simulink model "PID_discrete"  (R2019b)
settings: Solver=ode3  StartTime=0.0  StopTime=4  FixedStep=0.001  RelTol=1e-3
undefined symbols (not defined in the file): DiscIntNeverNeededParam
libraries: STLLib x15, discretizing x2
settings Model: Creator=balsi  LastModifiedBy=yuxia
settings DataIOCC: LimitDataPoints=on  SaveFormat=Array  ReturnWorkspaceOutputs=off
settings OptimizationCC: LifeSpan=inf
settings DebuggingCC: SFUnexpectedBacktrackingDiag=warning  SFNoUnconditionalDefaultTransitionDiag=warning  SFExecutionAtInitializationDiag=none  ArithmeticOperatorsInVariantConditions=warning
settings HardwareCC: ProdBitPerPointer=32  ProdBitPerSizeT=32  ProdBitPerPtrDiffT=32  ProdLargestAtomicFloat=None  ProdIntDivRoundTo=Undefined  ProdEndianess=Unspecified  ProdWordSize=32  ProdHWDeviceType=32-bit Generic
settings ModelReferenceCC: PropagateSignalLabelsOutOfModel=off
settings SFSimCC: SimUseLocalCustomCode=off  CustomCodeUndefinedFunction=UseInterfaceOnly
settings RTWCC: RTWUseLocalCustomCode=off
settings CodeAppCC: StateflowObjectComments=on
settings GRTTargetCC: TargetLangStandard=C89/C90 (ANSI)  GeneratePreprocessorConditionals=Disable all
settings ConfigComp: CovMetricSettings=dw  CovHtmlReporting=on  CovSaveCumulativeToWorkspaceVar=on  CovSaveSingleToWorkspaceVar=on  CovExternalEMLEnable=off

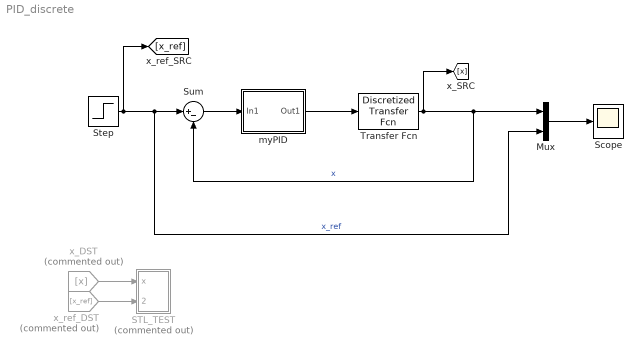
== system PID_discrete ==
  Mux : Mux  Inputs=2
  STL_TEST : Subsystem  Commented=on
  Scope : Scope
  Step : Step  After=10  SampleTime=0.01  mask(DiscretizedSource){}
      mask init:
      | %zoh
  Sum : Sum  Inputs=|+-
  Transfer Fcn : discretizing/Discretized Transfer Fcn  Numerator=[1]  Denominator=[1 1 1]  AbsTol=auto  SampleTime=0.01  method=zoh  Wc=1
      settings: SourceProductName=Simulink  SourceProductBaseCode=SL
  myPID : Subsystem
  x_DST : From  Commented=on  GotoTag=x
  x_ref_DST : From  Commented=on  GotoTag=x_ref
  wires:
  Step/1 -> Mux/2, Sum/1, [x_ref]  "x_ref"
  Mux/1 -> Scope/1
  myPID/1(Out1) -> Transfer Fcn/1
  Transfer Fcn/1 -> Mux/1, Sum/2, [x]  "x"
  Sum/1 -> myPID/1(In1)
  x_DST/1 -> STL_TEST/1(x)
  x_ref_DST/1 -> STL_TEST/2(x_ref)

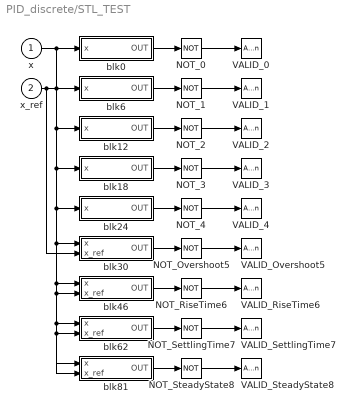
== system PID_discrete/STL_TEST ==
  x : Inport
  x_ref : Inport  Port=2
  NOT_{0..4} (5 alike) : Logic  Operator=NOT  AllPortsSameDT=off  OutDataTypeStr=boolean
  NOT_Overshoot5 : Logic  Operator=NOT  AllPortsSameDT=off  OutDataTypeStr=boolean
  NOT_RiseTime6 : Logic  Operator=NOT  AllPortsSameDT=off  OutDataTypeStr=boolean
  NOT_SettlingTime7 : Logic  Operator=NOT  AllPortsSameDT=off  OutDataTypeStr=boolean
  NOT_SteadyState8 : Logic  Operator=NOT  AllPortsSameDT=off  OutDataTypeStr=boolean
  VALID_{0..4} (5 alike) : Assertion
  VALID_Overshoot5 : Assertion
  VALID_RiseTime6 : Assertion
  VALID_SettlingTime7 : Assertion
  VALID_SteadyState8 : Assertion
  blk0 : Subsystem
  blk12 : Subsystem
  blk18 : Subsystem
  blk24 : Subsystem
  blk30 : Subsystem
  blk46 : Subsystem
  blk6 : Subsystem
  blk62 : Subsystem
  blk81 : Subsystem
  wires:
  NOT_0/1 -> VALID_0/1
  blk0/1(OUT) -> NOT_0/1
  x/1 -> blk62/1(x), blk81/1(x), blk46/1(x), blk30/1(x), blk24/1(x), blk18/1(x), blk12/1(x), blk6/1(x), blk0/1(x)
  NOT_1/1 -> VALID_1/1
  blk6/1(OUT) -> NOT_1/1
  NOT_2/1 -> VALID_2/1
  blk12/1(OUT) -> NOT_2/1
  NOT_3/1 -> VALID_3/1
  blk18/1(OUT) -> NOT_3/1
  NOT_4/1 -> VALID_4/1
  blk24/1(OUT) -> NOT_4/1
  NOT_Overshoot5/1 -> VALID_Overshoot5/1
  blk30/1(OUT) -> NOT_Overshoot5/1
  x_ref/1 -> blk62/2(x_ref), blk81/2(x_ref), blk46/2(x_ref), blk30/2(x_ref)
  NOT_RiseTime6/1 -> VALID_RiseTime6/1
  blk46/1(OUT) -> NOT_RiseTime6/1
  NOT_SettlingTime7/1 -> VALID_SettlingTime7/1
  blk62/1(OUT) -> NOT_SettlingTime7/1
  NOT_SteadyState8/1 -> VALID_SteadyState8/1
  blk81/1(OUT) -> NOT_SteadyState8/1

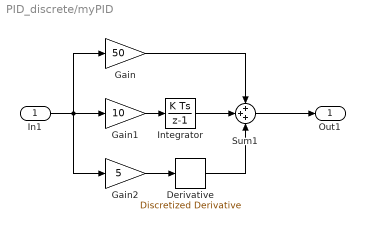
== system PID_discrete/myPID ==
  In1 : Inport
  Derivative : discretizing/Discretized Derivative  method=tustin  SampleTime=0.01  Wc=1
      settings: SourceProductName=Simulink  SourceProductBaseCode=SL
  Gain : Gain  Gain=50
  Gain1 : Gain  Gain=10
  Gain2 : Gain  Gain=5
  Integrator : DiscreteIntegrator  SampleTime=0.01  ICPrevOutput=DiscIntNeverNeededParam  ICPrevScaledInput=DiscIntNeverNeededParam  mask(DiscretizedDiscreteIntegrator){}
      mask init:
      | %zoh
  Sum1 : Sum  Inputs=+++
  Out1 : Outport
  wires:
  Derivative/1 -> Sum1/3
  Integrator/1 -> Sum1/2
  Gain/1 -> Sum1/1
  In1/1 -> Gain2/1, Gain/1, Gain1/1
  Sum1/1 -> Out1/1
  Gain1/1 -> Integrator/1
  Gain2/1 -> Derivative/1

== system PID_discrete/STL_TEST/blk0 ==
  x : Inport
  blk1 : Subsystem
  blk4 : Subsystem
  blk5 : Subsystem
  OUT : Outport
  wires:
  blk5/1(OUT) -> blk4/1(TIME)
  blk1/1(OUT) -> blk4/2(STL)
  blk4/1(OUT) -> OUT/1
  x/1 -> blk1/1(x)

== system PID_discrete/STL_TEST/blk12 ==
  x : Inport
  blk13 : Subsystem
  blk16 : Subsystem
  blk17 : Subsystem
  OUT : Outport
  wires:
  blk16/1(OUT) -> blk17/1(TIME)
  blk13/1(OUT) -> blk17/2(STL)
  blk17/1(OUT) -> OUT/1
  x/1 -> blk13/1(x)

== system PID_discrete/STL_TEST/blk18 ==
  x : Inport
  blk19 : Subsystem
  blk22 : Subsystem
  blk23 : Subsystem
  OUT : Outport
  wires:
  blk22/1(OUT) -> blk23/1(TIME)
  blk19/1(OUT) -> blk23/2(STL)
  blk23/1(OUT) -> OUT/1
  x/1 -> blk19/1(x)

== system PID_discrete/STL_TEST/blk24 ==
  x : Inport
  blk25 : Subsystem
  blk28 : Subsystem
  blk29 : Subsystem
  OUT : Outport
  wires:
  blk29/1(OUT) -> blk28/1(TIME)
  blk25/1(OUT) -> blk28/2(STL)
  blk28/1(OUT) -> OUT/1
  x/1 -> blk25/1(x)

== system PID_discrete/STL_TEST/blk30 ==
  x : Inport
  x_ref : Inport  Port=2
  blk31 : Subsystem
  blk44 : Subsystem
  blk45 : Subsystem
  OUT : Outport
  wires:
  blk44/1(OUT) -> blk45/1(TIME)
  blk31/1(OUT) -> blk45/2(STL)
  blk45/1(OUT) -> OUT/1
  x/1 -> blk31/1(x)
  x_ref/1 -> blk31/2(x_ref)

== system PID_discrete/STL_TEST/blk46 ==
  x : Inport
  x_ref : Inport  Port=2
  blk47 : Subsystem
  blk60 : Subsystem
  blk61 : Subsystem
  OUT : Outport
  wires:
  blk60/1(OUT) -> blk61/1(TIME)
  blk47/1(OUT) -> blk61/2(STL)
  blk61/1(OUT) -> OUT/1
  x/1 -> blk47/1(x)
  x_ref/1 -> blk47/2(x_ref)

== system PID_discrete/STL_TEST/blk6 ==
  x : Inport
  blk10 : Subsystem
  blk11 : Subsystem
  blk7 : Subsystem
  OUT : Outport
  wires:
  blk11/1(OUT) -> blk10/1(TIME)
  blk7/1(OUT) -> blk10/2(STL)
  blk10/1(OUT) -> OUT/1
  x/1 -> blk7/1(x)

== system PID_discrete/STL_TEST/blk62 ==
  x : Inport
  x_ref : Inport  Port=2
  blk63 : Subsystem
  blk79 : Subsystem
  blk80 : Subsystem
  OUT : Outport
  wires:
  blk79/1(OUT) -> blk80/1(TIME)
  blk63/1(OUT) -> blk80/2(STL)
  blk80/1(OUT) -> OUT/1
  x/1 -> blk63/1(x)
  x_ref/1 -> blk63/2(x_ref)

== system PID_discrete/STL_TEST/blk81 ==
  x : Inport
  x_ref : Inport  Port=2
  blk82 : Subsystem
  blk88 : Subsystem
  blk89 : Subsystem
  OUT : Outport
  wires:
  blk88/1(OUT) -> blk89/1(TIME)
  blk82/1(OUT) -> blk89/2(STL)
  blk89/1(OUT) -> OUT/1
  x/1 -> blk82/1(x)
  x_ref/1 -> blk82/2(x_ref)

== system PID_discrete/STL_TEST/blk0/blk1 ==
  x : Inport
  OP : RelationalOperator  Operator=>  OutDataTypeStr=boolean  RndMeth=Simplest
  blk2 : Subsystem
  blk3 : Subsystem
  OUT : Outport
  wires:
  OP/1 -> OUT/1
  blk2/1(OUT) -> OP/1
  blk3/1(OUT) -> OP/2
  x/1 -> blk2/1(x)

== system PID_discrete/STL_TEST/blk0/blk4 ==
  TIME : Inport
  STL : Inport  Port=2
  ALWAYS : STLLib/Always  SystemSampleTime=-1  Latency=0  AutoFrameSizeCalculation=off
  OUT : Outport
  wires:
  ALWAYS/1 -> OUT/1
  TIME/1 -> ALWAYS/2
  STL/1 -> ALWAYS/1

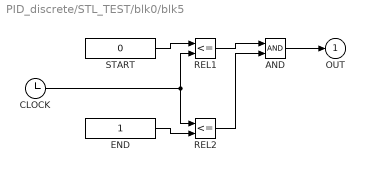
== system PID_discrete/STL_TEST/blk0/blk5 ==
  AND : Logic  AllPortsSameDT=off  OutDataTypeStr=boolean
  CLOCK : Clock
  END : Constant
  REL1 : RelationalOperator  Operator=<=  OutDataTypeStr=boolean  RndMeth=Simplest
  REL2 : RelationalOperator  Operator=<=  OutDataTypeStr=boolean  RndMeth=Simplest
  START : Constant  Value=0
  OUT : Outport
  wires:
  START/1 -> REL1/1
  CLOCK/1 -> REL1/2, REL2/1
  END/1 -> REL2/2
  REL1/1 -> AND/1
  REL2/1 -> AND/2
  AND/1 -> OUT/1

== system PID_discrete/STL_TEST/blk12/blk13 ==
  x : Inport
  OP : RelationalOperator  Operator=>  OutDataTypeStr=boolean  RndMeth=Simplest
  blk14 : Subsystem
  blk15 : Subsystem
  OUT : Outport
  wires:
  OP/1 -> OUT/1
  blk14/1(OUT) -> OP/1
  blk15/1(OUT) -> OP/2
  x/1 -> blk14/1(x)

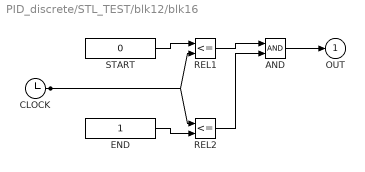
== system PID_discrete/STL_TEST/blk12/blk16 ==
  AND : Logic  AllPortsSameDT=off  OutDataTypeStr=boolean
  CLOCK : Clock
  END : Constant
  REL1 : RelationalOperator  Operator=<=  OutDataTypeStr=boolean  RndMeth=Simplest
  REL2 : RelationalOperator  Operator=<=  OutDataTypeStr=boolean  RndMeth=Simplest
  START : Constant  Value=0
  OUT : Outport
  wires:
  START/1 -> REL1/1
  CLOCK/1 -> REL1/2, REL2/1
  END/1 -> REL2/2
  REL1/1 -> AND/1
  REL2/1 -> AND/2
  AND/1 -> OUT/1

== system PID_discrete/STL_TEST/blk12/blk17 ==
  TIME : Inport
  STL : Inport  Port=2
  EVENTUALLY : STLLib/Eventually  SystemSampleTime=-1  Latency=0  AutoFrameSizeCalculation=off
  OUT : Outport
  wires:
  EVENTUALLY/1 -> OUT/1
  TIME/1 -> EVENTUALLY/2
  STL/1 -> EVENTUALLY/1

== system PID_discrete/STL_TEST/blk18/blk19 ==
  x : Inport
  OP : RelationalOperator  Operator===  OutDataTypeStr=boolean  RndMeth=Simplest
  blk20 : Subsystem
  blk21 : Subsystem
  OUT : Outport
  wires:
  OP/1 -> OUT/1
  blk20/1(OUT) -> OP/1
  blk21/1(OUT) -> OP/2
  x/1 -> blk20/1(x)

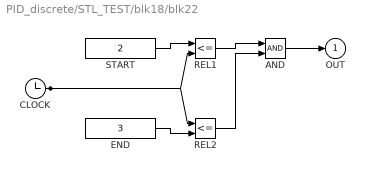
== system PID_discrete/STL_TEST/blk18/blk22 ==
  AND : Logic  AllPortsSameDT=off  OutDataTypeStr=boolean
  CLOCK : Clock
  END : Constant  Value=3
  REL1 : RelationalOperator  Operator=<=  OutDataTypeStr=boolean  RndMeth=Simplest
  REL2 : RelationalOperator  Operator=<=  OutDataTypeStr=boolean  RndMeth=Simplest
  START : Constant  Value=2
  OUT : Outport
  wires:
  START/1 -> REL1/1
  CLOCK/1 -> REL1/2, REL2/1
  END/1 -> REL2/2
  REL1/1 -> AND/1
  REL2/1 -> AND/2
  AND/1 -> OUT/1

== system PID_discrete/STL_TEST/blk18/blk23 ==
  TIME : Inport
  STL : Inport  Port=2
  EVENTUALLY : STLLib/Eventually  SystemSampleTime=-1  Latency=0  AutoFrameSizeCalculation=off
  OUT : Outport
  wires:
  EVENTUALLY/1 -> OUT/1
  TIME/1 -> EVENTUALLY/2
  STL/1 -> EVENTUALLY/1

== system PID_discrete/STL_TEST/blk24/blk25 ==
  x : Inport
  OP : RelationalOperator  Operator===  OutDataTypeStr=boolean  RndMeth=Simplest
  blk26 : Subsystem
  blk27 : Subsystem
  OUT : Outport
  wires:
  OP/1 -> OUT/1
  blk26/1(OUT) -> OP/1
  blk27/1(OUT) -> OP/2
  x/1 -> blk26/1(x)

== system PID_discrete/STL_TEST/blk24/blk28 ==
  TIME : Inport
  STL : Inport  Port=2
  ALWAYS : STLLib/Always  SystemSampleTime=-1  Latency=0  AutoFrameSizeCalculation=off
  OUT : Outport
  wires:
  ALWAYS/1 -> OUT/1
  TIME/1 -> ALWAYS/2
  STL/1 -> ALWAYS/1

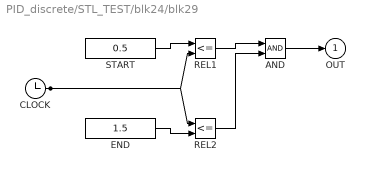
== system PID_discrete/STL_TEST/blk24/blk29 ==
  AND : Logic  AllPortsSameDT=off  OutDataTypeStr=boolean
  CLOCK : Clock
  END : Constant  Value=1.5
  REL1 : RelationalOperator  Operator=<=  OutDataTypeStr=boolean  RndMeth=Simplest
  REL2 : RelationalOperator  Operator=<=  OutDataTypeStr=boolean  RndMeth=Simplest
  START : Constant  Value=0.5
  OUT : Outport
  wires:
  START/1 -> REL1/1
  CLOCK/1 -> REL1/2, REL2/1
  END/1 -> REL2/2
  REL1/1 -> AND/1
  REL2/1 -> AND/2
  AND/1 -> OUT/1

== system PID_discrete/STL_TEST/blk30/blk31 ==
  x : Inport
  x_ref : Inport  Port=2
  ANDSTL : STLLib/ANDSTL  SystemSampleTime=-1  Latency=0  AutoFrameSizeCalculation=off
  blk32 : Subsystem
  blk36 : Subsystem
  OUT : Outport
  wires:
  ANDSTL/1 -> OUT/1
  blk32/1(OUT) -> ANDSTL/1
  blk36/1(OUT) -> ANDSTL/2
  x/1 -> blk36/1(x)
  x_ref/1 -> blk36/2(x_ref), blk32/1(x_ref)
  ANDSTL/2 -> blk36/3(REL_TIME)

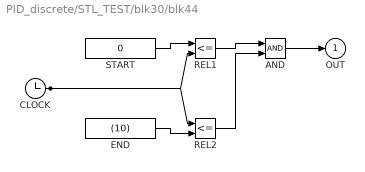
== system PID_discrete/STL_TEST/blk30/blk44 ==
  AND : Logic  AllPortsSameDT=off  OutDataTypeStr=boolean
  CLOCK : Clock
  END : Constant  Value=(10)
  REL1 : RelationalOperator  Operator=<=  OutDataTypeStr=boolean  RndMeth=Simplest
  REL2 : RelationalOperator  Operator=<=  OutDataTypeStr=boolean  RndMeth=Simplest
  START : Constant  Value=0
  OUT : Outport
  wires:
  START/1 -> REL1/1
  CLOCK/1 -> REL1/2, REL2/1
  END/1 -> REL2/2
  REL1/1 -> AND/1
  REL2/1 -> AND/2
  AND/1 -> OUT/1

== system PID_discrete/STL_TEST/blk30/blk45 ==
  TIME : Inport
  STL : Inport  Port=2
  EVENTUALLY : STLLib/Eventually  SystemSampleTime=-1  Latency=0  AutoFrameSizeCalculation=off
  OUT : Outport
  wires:
  EVENTUALLY/1 -> OUT/1
  TIME/1 -> EVENTUALLY/2
  STL/1 -> EVENTUALLY/1

== system PID_discrete/STL_TEST/blk46/blk47 ==
  x : Inport
  x_ref : Inport  Port=2
  ANDSTL : STLLib/ANDSTL  SystemSampleTime=-1  Latency=0  AutoFrameSizeCalculation=off
  blk48 : Subsystem
  blk52 : Subsystem
  OUT : Outport
  wires:
  ANDSTL/1 -> OUT/1
  blk48/1(OUT) -> ANDSTL/1
  blk52/1(OUT) -> ANDSTL/2
  x/1 -> blk52/1(x)
  x_ref/1 -> blk48/1(x_ref)
  ANDSTL/2 -> blk52/2(REL_TIME)

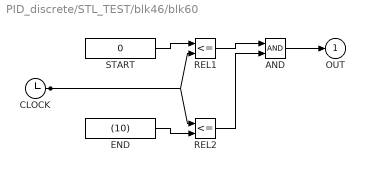
== system PID_discrete/STL_TEST/blk46/blk60 ==
  AND : Logic  AllPortsSameDT=off  OutDataTypeStr=boolean
  CLOCK : Clock
  END : Constant  Value=(10)
  REL1 : RelationalOperator  Operator=<=  OutDataTypeStr=boolean  RndMeth=Simplest
  REL2 : RelationalOperator  Operator=<=  OutDataTypeStr=boolean  RndMeth=Simplest
  START : Constant  Value=0
  OUT : Outport
  wires:
  START/1 -> REL1/1
  CLOCK/1 -> REL1/2, REL2/1
  END/1 -> REL2/2
  REL1/1 -> AND/1
  REL2/1 -> AND/2
  AND/1 -> OUT/1

== system PID_discrete/STL_TEST/blk46/blk61 ==
  TIME : Inport
  STL : Inport  Port=2
  EVENTUALLY : STLLib/Eventually  SystemSampleTime=-1  Latency=0  AutoFrameSizeCalculation=off
  OUT : Outport
  wires:
  EVENTUALLY/1 -> OUT/1
  TIME/1 -> EVENTUALLY/2
  STL/1 -> EVENTUALLY/1

== system PID_discrete/STL_TEST/blk6/blk10 ==
  TIME : Inport
  STL : Inport  Port=2
  ALWAYS : STLLib/Always  SystemSampleTime=-1  Latency=0  AutoFrameSizeCalculation=off
  OUT : Outport
  wires:
  ALWAYS/1 -> OUT/1
  TIME/1 -> ALWAYS/2
  STL/1 -> ALWAYS/1

== system PID_discrete/STL_TEST/blk6/blk11 ==
  AND : Logic  AllPortsSameDT=off  OutDataTypeStr=boolean
  CLOCK : Clock
  END : Constant  Value=5
  REL1 : RelationalOperator  Operator=<=  OutDataTypeStr=boolean  RndMeth=Simplest
  REL2 : RelationalOperator  Operator=<=  OutDataTypeStr=boolean  RndMeth=Simplest
  START : Constant  Value=0
  OUT : Outport
  wires:
  START/1 -> REL1/1
  CLOCK/1 -> REL1/2, REL2/1
  END/1 -> REL2/2
  REL1/1 -> AND/1
  REL2/1 -> AND/2
  AND/1 -> OUT/1

== system PID_discrete/STL_TEST/blk6/blk7 ==
  x : Inport
  OP : RelationalOperator  Operator=>  OutDataTypeStr=boolean  RndMeth=Simplest
  blk8 : Subsystem
  blk9 : Subsystem
  OUT : Outport
  wires:
  OP/1 -> OUT/1
  blk8/1(OUT) -> OP/1
  blk9/1(OUT) -> OP/2
  x/1 -> blk8/1(x)

== system PID_discrete/STL_TEST/blk62/blk63 ==
  x : Inport
  x_ref : Inport  Port=2
  ANDSTL : STLLib/ANDSTL  SystemSampleTime=-1  Latency=0  AutoFrameSizeCalculation=off
  blk64 : Subsystem
  blk68 : Subsystem
  OUT : Outport
  wires:
  ANDSTL/1 -> OUT/1
  blk64/1(OUT) -> ANDSTL/1
  blk68/1(OUT) -> ANDSTL/2
  x/1 -> blk68/1(x)
  x_ref/1 -> blk68/2(x_ref), blk64/1(x_ref)
  ANDSTL/2 -> blk68/3(REL_TIME)

== system PID_discrete/STL_TEST/blk62/blk79 ==
  AND : Logic  AllPortsSameDT=off  OutDataTypeStr=boolean
  CLOCK : Clock
  END : Constant  Value=(10)
  REL1 : RelationalOperator  Operator=<=  OutDataTypeStr=boolean  RndMeth=Simplest
  REL2 : RelationalOperator  Operator=<=  OutDataTypeStr=boolean  RndMeth=Simplest
  START : Constant  Value=0
  OUT : Outport
  wires:
  START/1 -> REL1/1
  CLOCK/1 -> REL1/2, REL2/1
  END/1 -> REL2/2
  REL1/1 -> AND/1
  REL2/1 -> AND/2
  AND/1 -> OUT/1

== system PID_discrete/STL_TEST/blk62/blk80 ==
  TIME : Inport
  STL : Inport  Port=2
  EVENTUALLY : STLLib/Eventually  SystemSampleTime=-1  Latency=0  AutoFrameSizeCalculation=off
  OUT : Outport
  wires:
  EVENTUALLY/1 -> OUT/1
  TIME/1 -> EVENTUALLY/2
  STL/1 -> EVENTUALLY/1

== system PID_discrete/STL_TEST/blk81/blk82 ==
  x : Inport
  x_ref : Inport  Port=2
  OP : RelationalOperator  Operator=>  OutDataTypeStr=boolean  RndMeth=Simplest
  blk83 : Subsystem
  blk87 : Subsystem
  OUT : Outport
  wires:
  OP/1 -> OUT/1
  blk83/1(OUT) -> OP/1
  blk87/1(OUT) -> OP/2
  x/1 -> blk83/1(x)
  x_ref/1 -> blk83/2(x_ref)

== system PID_discrete/STL_TEST/blk81/blk88 ==
  AND : Logic  AllPortsSameDT=off  OutDataTypeStr=boolean
  CLOCK : Clock
  END : Constant  Value=(10)
  REL1 : RelationalOperator  Operator=<=  OutDataTypeStr=boolean  RndMeth=Simplest
  REL2 : RelationalOperator  Operator=<=  OutDataTypeStr=boolean  RndMeth=Simplest
  START : Constant  Value=(10)
  OUT : Outport
  wires:
  START/1 -> REL1/1
  CLOCK/1 -> REL1/2, REL2/1
  END/1 -> REL2/2
  REL1/1 -> AND/1
  REL2/1 -> AND/2
  AND/1 -> OUT/1

== system PID_discrete/STL_TEST/blk81/blk89 ==
  TIME : Inport
  STL : Inport  Port=2
  EVENTUALLY : STLLib/Eventually  SystemSampleTime=-1  Latency=0  AutoFrameSizeCalculation=off
  OUT : Outport
  wires:
  EVENTUALLY/1 -> OUT/1
  TIME/1 -> EVENTUALLY/2
  STL/1 -> EVENTUALLY/1

== system PID_discrete/STL_TEST/blk0/blk1/blk2 ==
  x : Inport
  OUT : Outport
  wires:
  x/1 -> OUT/1

== system PID_discrete/STL_TEST/blk0/blk1/blk3 ==
  K : Constant
  OUT : Outport
  wires:
  K/1 -> OUT/1

== system PID_discrete/STL_TEST/blk12/blk13/blk14 ==
  x : Inport
  OUT : Outport
  wires:
  x/1 -> OUT/1

== system PID_discrete/STL_TEST/blk12/blk13/blk15 ==
  K : Constant
  OUT : Outport
  wires:
  K/1 -> OUT/1

== system PID_discrete/STL_TEST/blk18/blk19/blk20 ==
  x : Inport
  OUT : Outport
  wires:
  x/1 -> OUT/1

== system PID_discrete/STL_TEST/blk18/blk19/blk21 ==
  K : Constant  Value=0
  OUT : Outport
  wires:
  K/1 -> OUT/1

== system PID_discrete/STL_TEST/blk24/blk25/blk26 ==
  x : Inport
  OUT : Outport
  wires:
  x/1 -> OUT/1

== system PID_discrete/STL_TEST/blk24/blk25/blk27 ==
  K : Constant  Value=0
  OUT : Outport
  wires:
  K/1 -> OUT/1

== system PID_discrete/STL_TEST/blk30/blk31/blk32 ==
  x_ref : Inport
  blk33 : Subsystem
  blk34 : Subsystem
  blk35 : Subsystem
  OUT : Outport
  wires:
  blk35/1(OUT) -> OUT/1
  blk33/1(OUT) -> blk35/1(SIG)
  blk34/1(OUT) -> blk35/2(H)
  x_ref/1 -> blk33/1(x_ref)

== system PID_discrete/STL_TEST/blk30/blk31/blk36 ==
  x : Inport
  x_ref : Inport  Port=2
  REL_TIME : Inport  Port=3
  blk37 : Subsystem
  blk42 : Subsystem
  blk43 : Subsystem
  OUT : Outport
  wires:
  blk42/1(OUT) -> blk43/1(TIME)
  blk37/1(OUT) -> blk43/2(STL)
  blk43/1(OUT) -> OUT/1
  x/1 -> blk37/1(x)
  x_ref/1 -> blk37/2(x_ref)
  REL_TIME/1 -> blk42/1(DELAY)

== system PID_discrete/STL_TEST/blk46/blk47/blk48 ==
  x_ref : Inport
  blk49 : Subsystem
  blk50 : Subsystem
  blk51 : Subsystem
  OUT : Outport
  wires:
  blk51/1(OUT) -> OUT/1
  blk49/1(OUT) -> blk51/1(SIG)
  blk50/1(OUT) -> blk51/2(H)
  x_ref/1 -> blk49/1(x_ref)

== system PID_discrete/STL_TEST/blk46/blk47/blk52 ==
  x : Inport
  REL_TIME : Inport  Port=2
  blk53 : Subsystem
  blk58 : Subsystem
  blk59 : Subsystem
  OUT : Outport
  wires:
  blk59/1(OUT) -> blk58/1(TIME)
  blk53/1(OUT) -> blk58/2(STL)
  blk58/1(OUT) -> OUT/1
  x/1 -> blk53/1(x)
  REL_TIME/1 -> blk59/1(DELAY)

== system PID_discrete/STL_TEST/blk6/blk7/blk8 ==
  x : Inport
  OUT : Outport
  wires:
  x/1 -> OUT/1

== system PID_discrete/STL_TEST/blk6/blk7/blk9 ==
  K : Constant
  OUT : Outport
  wires:
  K/1 -> OUT/1

== system PID_discrete/STL_TEST/blk62/blk63/blk64 ==
  x_ref : Inport
  blk65 : Subsystem
  blk66 : Subsystem
  blk67 : Subsystem
  OUT : Outport
  wires:
  blk67/1(OUT) -> OUT/1
  blk65/1(OUT) -> blk67/1(SIG)
  blk66/1(OUT) -> blk67/2(H)
  x_ref/1 -> blk65/1(x_ref)

== system PID_discrete/STL_TEST/blk62/blk63/blk68 ==
  x : Inport
  x_ref : Inport  Port=2
  REL_TIME : Inport  Port=3
  blk69 : Subsystem
  blk77 : Subsystem
  blk78 : Subsystem
  OUT : Outport
  wires:
  blk77/1(OUT) -> blk78/1(TIME)
  blk69/1(OUT) -> blk78/2(STL)
  blk78/1(OUT) -> OUT/1
  x/1 -> blk69/1(x)
  x_ref/1 -> blk69/2(x_ref)
  REL_TIME/1 -> blk77/1(DELAY)

== system PID_discrete/STL_TEST/blk81/blk82/blk83 ==
  x : Inport
  x_ref : Inport  Port=2
  OP : Abs
  blk84 : Subsystem
  OUT : Outport
  wires:
  OP/1 -> OUT/1
  blk84/1(OUT) -> OP/1
  x/1 -> blk84/1(x)
  x_ref/1 -> blk84/2(x_ref)

== system PID_discrete/STL_TEST/blk81/blk82/blk87 ==
  K : Constant  Value=0.01
  OUT : Outport
  wires:
  K/1 -> OUT/1

== system PID_discrete/STL_TEST/blk30/blk31/blk32/blk33 ==
  x_ref : Inport
  OUT : Outport
  wires:
  x_ref/1 -> OUT/1

== system PID_discrete/STL_TEST/blk30/blk31/blk32/blk34 ==
  K : Constant  Value=5
  OUT : Outport
  wires:
  K/1 -> OUT/1

== system PID_discrete/STL_TEST/blk30/blk31/blk32/blk35 ==
  SIG : Inport
  H : Inport  Port=2
  CMP : RelationalOperator  Operator=>  OutDataTypeStr=boolean  RndMeth=Simplest
  MEM : Memory
  SUB : Sum  Inputs=+-
  OUT : Outport
  wires:
  SIG/1 -> MEM/1, SUB/1
  MEM/1 -> SUB/2
  SUB/1 -> CMP/1
  H/1 -> CMP/2
  CMP/1 -> OUT/1

== system PID_discrete/STL_TEST/blk30/blk31/blk36/blk37 ==
  x : Inport
  x_ref : Inport  Port=2
  OP : RelationalOperator  Operator=>  OutDataTypeStr=boolean  RndMeth=Simplest
  blk38 : Subsystem
  blk41 : Subsystem
  OUT : Outport
  wires:
  OP/1 -> OUT/1
  blk38/1(OUT) -> OP/1
  blk41/1(OUT) -> OP/2
  x/1 -> blk38/1(x)
  x_ref/1 -> blk38/2(x_ref)

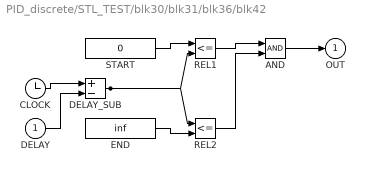
== system PID_discrete/STL_TEST/blk30/blk31/blk36/blk42 ==
  DELAY : Inport
  AND : Logic  AllPortsSameDT=off  OutDataTypeStr=boolean
  CLOCK : Clock
  DELAY_SUB : Sum  Inputs=+-
  END : Constant  Value=inf
  REL1 : RelationalOperator  Operator=<=  OutDataTypeStr=boolean  RndMeth=Simplest
  REL2 : RelationalOperator  Operator=<=  OutDataTypeStr=boolean  RndMeth=Simplest
  START : Constant  Value=0
  OUT : Outport
  wires:
  START/1 -> REL1/1
  DELAY/1 -> DELAY_SUB/2
  CLOCK/1 -> DELAY_SUB/1
  DELAY_SUB/1 -> REL1/2, REL2/1
  END/1 -> REL2/2
  REL1/1 -> AND/1
  REL2/1 -> AND/2
  AND/1 -> OUT/1

== system PID_discrete/STL_TEST/blk30/blk31/blk36/blk43 ==
  TIME : Inport
  STL : Inport  Port=2
  EVENTUALLY : STLLib/Eventually  SystemSampleTime=-1  Latency=0  AutoFrameSizeCalculation=off
  OUT : Outport
  wires:
  EVENTUALLY/1 -> OUT/1
  TIME/1 -> EVENTUALLY/2
  STL/1 -> EVENTUALLY/1

== system PID_discrete/STL_TEST/blk46/blk47/blk48/blk49 ==
  x_ref : Inport
  OUT : Outport
  wires:
  x_ref/1 -> OUT/1

== system PID_discrete/STL_TEST/blk46/blk47/blk48/blk50 ==
  K : Constant  Value=5
  OUT : Outport
  wires:
  K/1 -> OUT/1

== system PID_discrete/STL_TEST/blk46/blk47/blk48/blk51 ==
  SIG : Inport
  H : Inport  Port=2
  CMP : RelationalOperator  Operator=>  OutDataTypeStr=boolean  RndMeth=Simplest
  MEM : Memory
  SUB : Sum  Inputs=+-
  OUT : Outport
  wires:
  SIG/1 -> MEM/1, SUB/1
  MEM/1 -> SUB/2
  SUB/1 -> CMP/1
  H/1 -> CMP/2
  CMP/1 -> OUT/1

== system PID_discrete/STL_TEST/blk46/blk47/blk52/blk53 ==
  x : Inport
  OP : RelationalOperator  Operator=<  OutDataTypeStr=boolean  RndMeth=Simplest
  blk54 : Subsystem
  blk55 : Subsystem
  OUT : Outport
  wires:
  OP/1 -> OUT/1
  blk54/1(OUT) -> OP/1
  blk55/1(OUT) -> OP/2
  x/1 -> blk54/1(x)

== system PID_discrete/STL_TEST/blk46/blk47/blk52/blk58 ==
  TIME : Inport
  STL : Inport  Port=2
  ALWAYS : STLLib/Always  SystemSampleTime=-1  Latency=0  AutoFrameSizeCalculation=off
  OUT : Outport
  wires:
  ALWAYS/1 -> OUT/1
  TIME/1 -> ALWAYS/2
  STL/1 -> ALWAYS/1

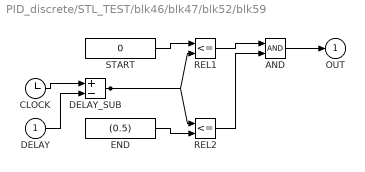
== system PID_discrete/STL_TEST/blk46/blk47/blk52/blk59 ==
  DELAY : Inport
  AND : Logic  AllPortsSameDT=off  OutDataTypeStr=boolean
  CLOCK : Clock
  DELAY_SUB : Sum  Inputs=+-
  END : Constant  Value=(0.5)
  REL1 : RelationalOperator  Operator=<=  OutDataTypeStr=boolean  RndMeth=Simplest
  REL2 : RelationalOperator  Operator=<=  OutDataTypeStr=boolean  RndMeth=Simplest
  START : Constant  Value=0
  OUT : Outport
  wires:
  START/1 -> REL1/1
  DELAY/1 -> DELAY_SUB/2
  CLOCK/1 -> DELAY_SUB/1
  DELAY_SUB/1 -> REL1/2, REL2/1
  END/1 -> REL2/2
  REL1/1 -> AND/1
  REL2/1 -> AND/2
  AND/1 -> OUT/1

== system PID_discrete/STL_TEST/blk62/blk63/blk64/blk65 ==
  x_ref : Inport
  OUT : Outport
  wires:
  x_ref/1 -> OUT/1

== system PID_discrete/STL_TEST/blk62/blk63/blk64/blk66 ==
  K : Constant  Value=5
  OUT : Outport
  wires:
  K/1 -> OUT/1

== system PID_discrete/STL_TEST/blk62/blk63/blk64/blk67 ==
  SIG : Inport
  H : Inport  Port=2
  CMP : RelationalOperator  Operator=>  OutDataTypeStr=boolean  RndMeth=Simplest
  MEM : Memory
  SUB : Sum  Inputs=+-
  OUT : Outport
  wires:
  SIG/1 -> MEM/1, SUB/1
  MEM/1 -> SUB/2
  SUB/1 -> CMP/1
  H/1 -> CMP/2
  CMP/1 -> OUT/1

== system PID_discrete/STL_TEST/blk62/blk63/blk68/blk69 ==
  x : Inport
  x_ref : Inport  Port=2
  OP : RelationalOperator  Operator=>  OutDataTypeStr=boolean  RndMeth=Simplest
  blk70 : Subsystem
  blk74 : Subsystem
  OUT : Outport
  wires:
  OP/1 -> OUT/1
  blk70/1(OUT) -> OP/1
  blk74/1(OUT) -> OP/2
  x/1 -> blk70/1(x)
  x_ref/1 -> blk70/2(x_ref), blk74/1(x_ref)

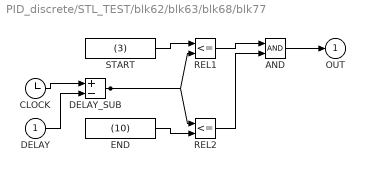
== system PID_discrete/STL_TEST/blk62/blk63/blk68/blk77 ==
  DELAY : Inport
  AND : Logic  AllPortsSameDT=off  OutDataTypeStr=boolean
  CLOCK : Clock
  DELAY_SUB : Sum  Inputs=+-
  END : Constant  Value=(10)
  REL1 : RelationalOperator  Operator=<=  OutDataTypeStr=boolean  RndMeth=Simplest
  REL2 : RelationalOperator  Operator=<=  OutDataTypeStr=boolean  RndMeth=Simplest
  START : Constant  Value=(3)
  OUT : Outport
  wires:
  START/1 -> REL1/1
  DELAY/1 -> DELAY_SUB/2
  CLOCK/1 -> DELAY_SUB/1
  DELAY_SUB/1 -> REL1/2, REL2/1
  END/1 -> REL2/2
  REL1/1 -> AND/1
  REL2/1 -> AND/2
  AND/1 -> OUT/1

== system PID_discrete/STL_TEST/blk62/blk63/blk68/blk78 ==
  TIME : Inport
  STL : Inport  Port=2
  EVENTUALLY : STLLib/Eventually  SystemSampleTime=-1  Latency=0  AutoFrameSizeCalculation=off
  OUT : Outport
  wires:
  EVENTUALLY/1 -> OUT/1
  TIME/1 -> EVENTUALLY/2
  STL/1 -> EVENTUALLY/1

== system PID_discrete/STL_TEST/blk81/blk82/blk83/blk84 ==
  x : Inport
  x_ref : Inport  Port=2
  OP : Sum  Inputs=+-
  blk85 : Subsystem
  blk86 : Subsystem
  OUT : Outport
  wires:
  OP/1 -> OUT/1
  blk85/1(OUT) -> OP/1
  blk86/1(OUT) -> OP/2
  x/1 -> blk85/1(x)
  x_ref/1 -> blk86/1(x_ref)

== system PID_discrete/STL_TEST/blk30/blk31/blk36/blk37/blk38 ==
  x : Inport
  x_ref : Inport  Port=2
  OP : Sum  Inputs=+-
  blk39 : Subsystem
  blk40 : Subsystem
  OUT : Outport
  wires:
  OP/1 -> OUT/1
  blk39/1(OUT) -> OP/1
  blk40/1(OUT) -> OP/2
  x/1 -> blk39/1(x)
  x_ref/1 -> blk40/1(x_ref)

== system PID_discrete/STL_TEST/blk30/blk31/blk36/blk37/blk41 ==
  K : Constant  Value=3
  OUT : Outport
  wires:
  K/1 -> OUT/1

== system PID_discrete/STL_TEST/blk46/blk47/blk52/blk53/blk54 ==
  x : Inport
  OUT : Outport
  wires:
  x/1 -> OUT/1

== system PID_discrete/STL_TEST/blk46/blk47/blk52/blk53/blk55 ==
  OP : Product
  blk56 : Subsystem
  blk57 : Subsystem
  OUT : Outport
  wires:
  OP/1 -> OUT/1
  blk56/1(OUT) -> OP/1
  blk57/1(OUT) -> OP/2

== system PID_discrete/STL_TEST/blk62/blk63/blk68/blk69/blk70 ==
  x : Inport
  x_ref : Inport  Port=2
  OP : Abs
  blk71 : Subsystem
  OUT : Outport
  wires:
  OP/1 -> OUT/1
  blk71/1(OUT) -> OP/1
  x/1 -> blk71/1(x)
  x_ref/1 -> blk71/2(x_ref)

== system PID_discrete/STL_TEST/blk62/blk63/blk68/blk69/blk74 ==
  x_ref : Inport
  OP : Product
  blk75 : Subsystem
  blk76 : Subsystem
  OUT : Outport
  wires:
  OP/1 -> OUT/1
  blk75/1(OUT) -> OP/1
  blk76/1(OUT) -> OP/2
  x_ref/1 -> blk76/1(x_ref)

== system PID_discrete/STL_TEST/blk81/blk82/blk83/blk84/blk85 ==
  x : Inport
  OUT : Outport
  wires:
  x/1 -> OUT/1

== system PID_discrete/STL_TEST/blk81/blk82/blk83/blk84/blk86 ==
  x_ref : Inport
  OUT : Outport
  wires:
  x_ref/1 -> OUT/1

== system PID_discrete/STL_TEST/blk30/blk31/blk36/blk37/blk38/blk39 ==
  x : Inport
  OUT : Outport
  wires:
  x/1 -> OUT/1

== system PID_discrete/STL_TEST/blk30/blk31/blk36/blk37/blk38/blk40 ==
  x_ref : Inport
  OUT : Outport
  wires:
  x_ref/1 -> OUT/1

== system PID_discrete/STL_TEST/blk46/blk47/blk52/blk53/blk55/blk56 ==
  K : Constant  Value=0.95
  OUT : Outport
  wires:
  K/1 -> OUT/1

== system PID_discrete/STL_TEST/blk46/blk47/blk52/blk53/blk55/blk57 ==
  K : Constant  Value=10
  OUT : Outport
  wires:
  K/1 -> OUT/1

== system PID_discrete/STL_TEST/blk62/blk63/blk68/blk69/blk70/blk71 ==
  x : Inport
  x_ref : Inport  Port=2
  OP : Sum  Inputs=+-
  blk72 : Subsystem
  blk73 : Subsystem
  OUT : Outport
  wires:
  OP/1 -> OUT/1
  blk72/1(OUT) -> OP/1
  blk73/1(OUT) -> OP/2
  x/1 -> blk72/1(x)
  x_ref/1 -> blk73/1(x_ref)

== system PID_discrete/STL_TEST/blk62/blk63/blk68/blk69/blk74/blk75 ==
  K : Constant  Value=0.02
  OUT : Outport
  wires:
  K/1 -> OUT/1

== system PID_discrete/STL_TEST/blk62/blk63/blk68/blk69/blk74/blk76 ==
  x_ref : Inport
  OUT : Outport
  wires:
  x_ref/1 -> OUT/1

== system PID_discrete/STL_TEST/blk62/blk63/blk68/blk69/blk70/blk71/blk72 ==
  x : Inport
  OUT : Outport
  wires:
  x/1 -> OUT/1

== system PID_discrete/STL_TEST/blk62/blk63/blk68/blk69/blk70/blk71/blk73 ==
  x_ref : Inport
  OUT : Outport
  wires:
  x_ref/1 -> OUT/1
